simulink model "building_PHPP_v2"  (R2023b)
settings: Solver=ode23s  StartTime=-building.preruntime+8760*3600  StopTime=building.runtime+8760*3600  EnableMultiTasking=on
PreLoadFcn:
  | tic
StartFcn:
  | pre_time = toc
  | assignin('base','pre_time',pre_time)
  | tic
StopFcn:
  | time = toc
  | assignin('base','time',time)
values from neighbouring files (symbols this model uses):
  building = obj    [BUILDING.m]    (also in create_building_automatic.m = building.save(); ini_building_automatic.m = building.add_variant_hvac(building.variant_hvac, hvac); load_building_automatic.m = building.save())
  cp = str2num(value)    [CONSTRUCTION.m]
  p = [timevec_weather weather(:,12)]    [BOUNDARY.m]    (also in WEATHER.m = 0; init_carnotUIBK.m = cell2mat(carnotUIBKpaths(i,2)))
  rho = str2num(value)    [CONSTRUCTION.m]    (also in theta_ground_v1.m = 2000)
undefined symbols (not defined in the file or in its folder): Dreifach, get_building, Qdot_C, Qdot_C_energy, Qdot_H, Qdot_H_energy, Qdot_I_electricity, Qdot_I_electricity_energy, Qdot_I_light, Qdot_I_light_energy, Qdot_I_person, Qdot_I_person_energy, Qdot_S, Qdot_S_energy, Qdot_T_ground, Qdot_T_ground_energy, Qdot_T_neighbour, Qdot_T_neighbour_energy, Qdot_T_opaque, Qdot_T_opaque_energy, Qdot_T_window, Qdot_T_window_energy, Qdot_V_infiltration, Qdot_V_infiltration_energy, Qdot_V_mech, Qdot_V_mech_energy, Qdot_V_window, Qdot_V_window_energy, Tc, Tr, Ts, Wärmeschutzglas, x_CO2, x_H2O, x_VOC
libraries: carnotUIBK x2418, carnot x1
(part 31 of 32)

== system building_PHPP_v2/DATALOGGER/logger_BDB/z1 ==
  BDB : Inport
  Bus Assignment : BusAssignment  AssignedSignals=Qdot_T_opaque_energy,Qdot_T_ground_energy,Qdot_T_neighbour_energy,Qdot_T_window_energy,Qdot_V_mech_energy,Qdot_V_window_energy,Qdot_V_infiltration_energy,Qdot_S_energy,Qdot_I_person_energy,Qdot_I_light_energy,Qdot_I_electricity_energy,Qdot_H_energy,Qdot_C_energy
  Bus Creator1 : BusCreator  Inputs=13
  Bus Selector1 : BusSelector  OutputSignals=z1.Qdot_T_opaque,z1.Qdot_T_ground,z1.Qdot_T_neighbour,z1.Qdot_T_window,z1.Qdot_V_mech,z1.Qdot_V_window,z1.Qdot_V_infiltration,z1.Qdot_S,z1.Qdot_I_person,z1.Qdot_I_light,z1.Qdot_I_electricity,z1.Qdot_H,z1.Qdot_C
  Constant{,1..12} (13 alike) : Constant  Value=0
  Subsystem : Subsystem
  Subsystem1 : Subsystem
  Subsystem10 : Subsystem
  Subsystem11 : Subsystem
  Subsystem12 : Subsystem
  Subsystem2 : Subsystem
  Subsystem3 : Subsystem
  Subsystem4 : Subsystem
  Subsystem5 : Subsystem
  Subsystem6 : Subsystem
  Subsystem7 : Subsystem
  Subsystem8 : Subsystem
  Subsystem9 : Subsystem
  BDBenergy : Outport  VectorParamsAs1DForOutWhenUnconnected=off
  wires:
  Constant12/1 -> Bus Creator1/13  "Qdot_C_energy"
  Constant2/1 -> Bus Creator1/3  "Qdot_T_neighbour_energy"
  Constant4/1 -> Bus Creator1/5  "Qdot_V_mech_energy"
  Constant9/1 -> Bus Creator1/10  "Qdot_I_light_energy"
  Constant1/1 -> Bus Creator1/2  "Qdot_T_ground_energy"
  Constant3/1 -> Bus Creator1/4  "Qdot_T_window_energy"
  Constant11/1 -> Bus Creator1/12  "Qdot_H_energy"
  Constant10/1 -> Bus Creator1/11  "Qdot_I_electricity_energy"
  Constant/1 -> Bus Creator1/1  "Qdot_T_opaque_energy"
  Constant8/1 -> Bus Creator1/8  "Qdot_S_energy"
  Constant7/1 -> Bus Creator1/9  "Qdot_I_person_energy"
  Constant6/1 -> Bus Creator1/7  "Qdot_V_infiltration_energy"
  BDB/1 -> Bus Selector1/1
  Constant5/1 -> Bus Creator1/6  "Qdot_V_window_energy"
  Bus Selector1/1 -> Subsystem/1(In1)  "<Qdot_T_opaque>"
  Bus Selector1/4 -> Subsystem3/1(In1)  "<Qdot_T_window>"
  Bus Selector1/3 -> Subsystem2/1(In1)  "<Qdot_T_neighbour>"
  Bus Selector1/2 -> Subsystem1/1(In1)  "<Qdot_T_ground>"
  Bus Selector1/9 -> Subsystem8/1(In1)  "<Qdot_I_person>"
  Bus Selector1/10 -> Subsystem9/1(In1)  "<Qdot_I_light>"
  Bus Selector1/11 -> Subsystem10/1(In1)  "<Qdot_I_electricity>"
  Bus Selector1/12 -> Subsystem11/1(In1)  "<Qdot_H>"
  Bus Selector1/13 -> Subsystem12/1(In1)  "<Qdot_C>"
  Bus Selector1/8 -> Subsystem7/1(In1)  "<Qdot_S>"
  Bus Selector1/7 -> Subsystem6/1(In1)  "<Qdot_V_infiltration>"
  Bus Selector1/6 -> Subsystem5/1(In1)  "<Qdot_V_window>"
  Bus Selector1/5 -> Subsystem4/1(In1)  "<Qdot_V_mech>"
  Bus Assignment/1 -> BDBenergy/1
  Bus Creator1/1 -> Bus Assignment/1
  Subsystem/1(Out1) -> Bus Assignment/2
  Subsystem12/1(Out1) -> Bus Assignment/14
  Subsystem11/1(Out1) -> Bus Assignment/13
  Subsystem10/1(Out1) -> Bus Assignment/12
  Subsystem9/1(Out1) -> Bus Assignment/11
  Subsystem8/1(Out1) -> Bus Assignment/10
  Subsystem7/1(Out1) -> Bus Assignment/9
  Subsystem6/1(Out1) -> Bus Assignment/8
  Subsystem5/1(Out1) -> Bus Assignment/7
  Subsystem4/1(Out1) -> Bus Assignment/6
  Subsystem3/1(Out1) -> Bus Assignment/5
  Subsystem2/1(Out1) -> Bus Assignment/4
  Subsystem1/1(Out1) -> Bus Assignment/3

== system building_PHPP_v2/DATALOGGER/logger_BDB/z10 ==
  BDB : Inport
  Bus Assignment : BusAssignment  AssignedSignals=Qdot_T_opaque_energy,Qdot_T_ground_energy,Qdot_T_neighbour_energy,Qdot_T_window_energy,Qdot_V_mech_energy,Qdot_V_window_energy,Qdot_V_infiltration_energy,Qdot_S_energy,Qdot_I_person_energy,Qdot_I_light_energy,Qdot_I_electricity_energy,Qdot_H_energy,Qdot_C_energy
  Bus Creator1 : BusCreator  Inputs=13
  Bus Selector1 : BusSelector  OutputSignals=z10.Qdot_T_opaque,z10.Qdot_T_ground,z10.Qdot_T_neighbour,z10.Qdot_T_window,z10.Qdot_V_mech,z10.Qdot_V_window,z10.Qdot_V_infiltration,z10.Qdot_S,z10.Qdot_I_person,z10.Qdot_I_light,z10.Qdot_I_electricity,z10.Qdot_H,z10.Qdot_C
  Constant{,1..12} (13 alike) : Constant  Value=0
  Subsystem : Subsystem
  Subsystem1 : Subsystem
  Subsystem10 : Subsystem
  Subsystem11 : Subsystem
  Subsystem12 : Subsystem
  Subsystem2 : Subsystem
  Subsystem3 : Subsystem
  Subsystem4 : Subsystem
  Subsystem5 : Subsystem
  Subsystem6 : Subsystem
  Subsystem7 : Subsystem
  Subsystem8 : Subsystem
  Subsystem9 : Subsystem
  BDBenergy : Outport  VectorParamsAs1DForOutWhenUnconnected=off
  wires:
  Subsystem1/1(Out1) -> Bus Assignment/3
  Subsystem2/1(Out1) -> Bus Assignment/4
  Subsystem3/1(Out1) -> Bus Assignment/5
  Subsystem4/1(Out1) -> Bus Assignment/6
  Subsystem5/1(Out1) -> Bus Assignment/7
  Subsystem6/1(Out1) -> Bus Assignment/8
  Subsystem7/1(Out1) -> Bus Assignment/9
  Subsystem8/1(Out1) -> Bus Assignment/10
  Subsystem9/1(Out1) -> Bus Assignment/11
  Subsystem10/1(Out1) -> Bus Assignment/12
  Subsystem11/1(Out1) -> Bus Assignment/13
  Subsystem12/1(Out1) -> Bus Assignment/14
  Subsystem/1(Out1) -> Bus Assignment/2
  Bus Creator1/1 -> Bus Assignment/1
  Bus Assignment/1 -> BDBenergy/1
  Bus Selector1/5 -> Subsystem4/1(In1)  "<Qdot_V_mech>"
  Bus Selector1/6 -> Subsystem5/1(In1)  "<Qdot_V_window>"
  Bus Selector1/7 -> Subsystem6/1(In1)  "<Qdot_V_infiltration>"
  Bus Selector1/8 -> Subsystem7/1(In1)  "<Qdot_S>"
  Bus Selector1/13 -> Subsystem12/1(In1)  "<Qdot_C>"
  Bus Selector1/12 -> Subsystem11/1(In1)  "<Qdot_H>"
  Bus Selector1/11 -> Subsystem10/1(In1)  "<Qdot_I_electricity>"
  Bus Selector1/10 -> Subsystem9/1(In1)  "<Qdot_I_light>"
  Bus Selector1/9 -> Subsystem8/1(In1)  "<Qdot_I_person>"
  Bus Selector1/2 -> Subsystem1/1(In1)  "<Qdot_T_ground>"
  Bus Selector1/3 -> Subsystem2/1(In1)  "<Qdot_T_neighbour>"
  Bus Selector1/4 -> Subsystem3/1(In1)  "<Qdot_T_window>"
  Bus Selector1/1 -> Subsystem/1(In1)  "<Qdot_T_opaque>"
  Constant5/1 -> Bus Creator1/6  "Qdot_V_window_energy"
  BDB/1 -> Bus Selector1/1
  Constant6/1 -> Bus Creator1/7  "Qdot_V_infiltration_energy"
  Constant7/1 -> Bus Creator1/9  "Qdot_I_person_energy"
  Constant8/1 -> Bus Creator1/8  "Qdot_S_energy"
  Constant/1 -> Bus Creator1/1  "Qdot_T_opaque_energy"
  Constant10/1 -> Bus Creator1/11  "Qdot_I_electricity_energy"
  Constant11/1 -> Bus Creator1/12  "Qdot_H_energy"
  Constant3/1 -> Bus Creator1/4  "Qdot_T_window_energy"
  Constant1/1 -> Bus Creator1/2  "Qdot_T_ground_energy"
  Constant9/1 -> Bus Creator1/10  "Qdot_I_light_energy"
  Constant4/1 -> Bus Creator1/5  "Qdot_V_mech_energy"
  Constant2/1 -> Bus Creator1/3  "Qdot_T_neighbour_energy"
  Constant12/1 -> Bus Creator1/13  "Qdot_C_energy"

== system building_PHPP_v2/DATALOGGER/logger_BDB/z2 ==
  BDB : Inport
  Bus Assignment : BusAssignment  AssignedSignals=Qdot_T_opaque_energy,Qdot_T_ground_energy,Qdot_T_neighbour_energy,Qdot_T_window_energy,Qdot_V_mech_energy,Qdot_V_window_energy,Qdot_V_infiltration_energy,Qdot_S_energy,Qdot_I_person_energy,Qdot_I_light_energy,Qdot_I_electricity_energy,Qdot_H_energy,Qdot_C_energy
  Bus Creator1 : BusCreator  Inputs=13
  Bus Selector1 : BusSelector  OutputSignals=z2.Qdot_T_opaque,z2.Qdot_T_ground,z2.Qdot_T_neighbour,z2.Qdot_T_window,z2.Qdot_V_mech,z2.Qdot_V_window,z2.Qdot_V_infiltration,z2.Qdot_S,z2.Qdot_I_person,z2.Qdot_I_light,z2.Qdot_I_electricity,z2.Qdot_H,z2.Qdot_C
  Constant{,1..12} (13 alike) : Constant  Value=0
  Subsystem : Subsystem
  Subsystem1 : Subsystem
  Subsystem10 : Subsystem
  Subsystem11 : Subsystem
  Subsystem12 : Subsystem
  Subsystem2 : Subsystem
  Subsystem3 : Subsystem
  Subsystem4 : Subsystem
  Subsystem5 : Subsystem
  Subsystem6 : Subsystem
  Subsystem7 : Subsystem
  Subsystem8 : Subsystem
  Subsystem9 : Subsystem
  BDBenergy : Outport  VectorParamsAs1DForOutWhenUnconnected=off
  wires:
  Subsystem1/1(Out1) -> Bus Assignment/3
  Subsystem2/1(Out1) -> Bus Assignment/4
  Subsystem3/1(Out1) -> Bus Assignment/5
  Subsystem4/1(Out1) -> Bus Assignment/6
  Subsystem5/1(Out1) -> Bus Assignment/7
  Subsystem6/1(Out1) -> Bus Assignment/8
  Subsystem7/1(Out1) -> Bus Assignment/9
  Subsystem8/1(Out1) -> Bus Assignment/10
  Subsystem9/1(Out1) -> Bus Assignment/11
  Subsystem10/1(Out1) -> Bus Assignment/12
  Subsystem11/1(Out1) -> Bus Assignment/13
  Subsystem12/1(Out1) -> Bus Assignment/14
  Subsystem/1(Out1) -> Bus Assignment/2
  Bus Creator1/1 -> Bus Assignment/1
  Bus Assignment/1 -> BDBenergy/1
  Bus Selector1/5 -> Subsystem4/1(In1)  "<Qdot_V_mech>"
  Bus Selector1/6 -> Subsystem5/1(In1)  "<Qdot_V_window>"
  Bus Selector1/7 -> Subsystem6/1(In1)  "<Qdot_V_infiltration>"
  Bus Selector1/8 -> Subsystem7/1(In1)  "<Qdot_S>"
  Bus Selector1/13 -> Subsystem12/1(In1)  "<Qdot_C>"
  Bus Selector1/12 -> Subsystem11/1(In1)  "<Qdot_H>"
  Bus Selector1/11 -> Subsystem10/1(In1)  "<Qdot_I_electricity>"
  Bus Selector1/10 -> Subsystem9/1(In1)  "<Qdot_I_light>"
  Bus Selector1/9 -> Subsystem8/1(In1)  "<Qdot_I_person>"
  Bus Selector1/2 -> Subsystem1/1(In1)  "<Qdot_T_ground>"
  Bus Selector1/3 -> Subsystem2/1(In1)  "<Qdot_T_neighbour>"
  Bus Selector1/4 -> Subsystem3/1(In1)  "<Qdot_T_window>"
  Bus Selector1/1 -> Subsystem/1(In1)  "<Qdot_T_opaque>"
  Constant5/1 -> Bus Creator1/6  "Qdot_V_window_energy"
  BDB/1 -> Bus Selector1/1
  Constant6/1 -> Bus Creator1/7  "Qdot_V_infiltration_energy"
  Constant7/1 -> Bus Creator1/9  "Qdot_I_person_energy"
  Constant8/1 -> Bus Creator1/8  "Qdot_S_energy"
  Constant/1 -> Bus Creator1/1  "Qdot_T_opaque_energy"
  Constant10/1 -> Bus Creator1/11  "Qdot_I_electricity_energy"
  Constant11/1 -> Bus Creator1/12  "Qdot_H_energy"
  Constant3/1 -> Bus Creator1/4  "Qdot_T_window_energy"
  Constant1/1 -> Bus Creator1/2  "Qdot_T_ground_energy"
  Constant9/1 -> Bus Creator1/10  "Qdot_I_light_energy"
  Constant4/1 -> Bus Creator1/5  "Qdot_V_mech_energy"
  Constant2/1 -> Bus Creator1/3  "Qdot_T_neighbour_energy"
  Constant12/1 -> Bus Creator1/13  "Qdot_C_energy"

== system building_PHPP_v2/DATALOGGER/logger_BDB/z3 ==
  BDB : Inport
  Bus Assignment : BusAssignment  AssignedSignals=Qdot_T_opaque_energy,Qdot_T_ground_energy,Qdot_T_neighbour_energy,Qdot_T_window_energy,Qdot_V_mech_energy,Qdot_V_window_energy,Qdot_V_infiltration_energy,Qdot_S_energy,Qdot_I_person_energy,Qdot_I_light_energy,Qdot_I_electricity_energy,Qdot_H_energy,Qdot_C_energy
  Bus Creator1 : BusCreator  Inputs=13
  Bus Selector1 : BusSelector  OutputSignals=z3.Qdot_T_opaque,z3.Qdot_T_ground,z3.Qdot_T_neighbour,z3.Qdot_T_window,z3.Qdot_V_mech,z3.Qdot_V_window,z3.Qdot_V_infiltration,z3.Qdot_S,z3.Qdot_I_person,z3.Qdot_I_light,z3.Qdot_I_electricity,z3.Qdot_H,z3.Qdot_C
  Constant{,1..12} (13 alike) : Constant  Value=0
  Subsystem : Subsystem
  Subsystem1 : Subsystem
  Subsystem10 : Subsystem
  Subsystem11 : Subsystem
  Subsystem12 : Subsystem
  Subsystem2 : Subsystem
  Subsystem3 : Subsystem
  Subsystem4 : Subsystem
  Subsystem5 : Subsystem
  Subsystem6 : Subsystem
  Subsystem7 : Subsystem
  Subsystem8 : Subsystem
  Subsystem9 : Subsystem
  BDBenergy : Outport  VectorParamsAs1DForOutWhenUnconnected=off
  wires:
  Constant12/1 -> Bus Creator1/13  "Qdot_C_energy"
  Constant2/1 -> Bus Creator1/3  "Qdot_T_neighbour_energy"
  Constant4/1 -> Bus Creator1/5  "Qdot_V_mech_energy"
  Constant9/1 -> Bus Creator1/10  "Qdot_I_light_energy"
  Constant1/1 -> Bus Creator1/2  "Qdot_T_ground_energy"
  Constant3/1 -> Bus Creator1/4  "Qdot_T_window_energy"
  Constant11/1 -> Bus Creator1/12  "Qdot_H_energy"
  Constant10/1 -> Bus Creator1/11  "Qdot_I_electricity_energy"
  Constant/1 -> Bus Creator1/1  "Qdot_T_opaque_energy"
  Constant8/1 -> Bus Creator1/8  "Qdot_S_energy"
  Constant7/1 -> Bus Creator1/9  "Qdot_I_person_energy"
  Constant6/1 -> Bus Creator1/7  "Qdot_V_infiltration_energy"
  BDB/1 -> Bus Selector1/1
  Constant5/1 -> Bus Creator1/6  "Qdot_V_window_energy"
  Bus Selector1/1 -> Subsystem/1(In1)  "<Qdot_T_opaque>"
  Bus Selector1/4 -> Subsystem3/1(In1)  "<Qdot_T_window>"
  Bus Selector1/3 -> Subsystem2/1(In1)  "<Qdot_T_neighbour>"
  Bus Selector1/2 -> Subsystem1/1(In1)  "<Qdot_T_ground>"
  Bus Selector1/9 -> Subsystem8/1(In1)  "<Qdot_I_person>"
  Bus Selector1/10 -> Subsystem9/1(In1)  "<Qdot_I_light>"
  Bus Selector1/11 -> Subsystem10/1(In1)  "<Qdot_I_electricity>"
  Bus Selector1/12 -> Subsystem11/1(In1)  "<Qdot_H>"
  Bus Selector1/13 -> Subsystem12/1(In1)  "<Qdot_C>"
  Bus Selector1/8 -> Subsystem7/1(In1)  "<Qdot_S>"
  Bus Selector1/7 -> Subsystem6/1(In1)  "<Qdot_V_infiltration>"
  Bus Selector1/6 -> Subsystem5/1(In1)  "<Qdot_V_window>"
  Bus Selector1/5 -> Subsystem4/1(In1)  "<Qdot_V_mech>"
  Bus Assignment/1 -> BDBenergy/1
  Bus Creator1/1 -> Bus Assignment/1
  Subsystem/1(Out1) -> Bus Assignment/2
  Subsystem12/1(Out1) -> Bus Assignment/14
  Subsystem11/1(Out1) -> Bus Assignment/13
  Subsystem10/1(Out1) -> Bus Assignment/12
  Subsystem9/1(Out1) -> Bus Assignment/11
  Subsystem8/1(Out1) -> Bus Assignment/10
  Subsystem7/1(Out1) -> Bus Assignment/9
  Subsystem6/1(Out1) -> Bus Assignment/8
  Subsystem5/1(Out1) -> Bus Assignment/7
  Subsystem4/1(Out1) -> Bus Assignment/6
  Subsystem3/1(Out1) -> Bus Assignment/5
  Subsystem2/1(Out1) -> Bus Assignment/4
  Subsystem1/1(Out1) -> Bus Assignment/3

== system building_PHPP_v2/DATALOGGER/logger_BDB/z4 ==
  BDB : Inport
  Bus Assignment : BusAssignment  AssignedSignals=Qdot_T_opaque_energy,Qdot_T_ground_energy,Qdot_T_neighbour_energy,Qdot_T_window_energy,Qdot_V_mech_energy,Qdot_V_window_energy,Qdot_V_infiltration_energy,Qdot_S_energy,Qdot_I_person_energy,Qdot_I_light_energy,Qdot_I_electricity_energy,Qdot_H_energy,Qdot_C_energy
  Bus Creator1 : BusCreator  Inputs=13
  Bus Selector1 : BusSelector  OutputSignals=z4.Qdot_T_opaque,z4.Qdot_T_ground,z4.Qdot_T_neighbour,z4.Qdot_T_window,z4.Qdot_V_mech,z4.Qdot_V_window,z4.Qdot_V_infiltration,z4.Qdot_S,z4.Qdot_I_person,z4.Qdot_I_light,z4.Qdot_I_electricity,z4.Qdot_H,z4.Qdot_C
  Constant{,1..12} (13 alike) : Constant  Value=0
  Subsystem : Subsystem
  Subsystem1 : Subsystem
  Subsystem10 : Subsystem
  Subsystem11 : Subsystem
  Subsystem12 : Subsystem
  Subsystem2 : Subsystem
  Subsystem3 : Subsystem
  Subsystem4 : Subsystem
  Subsystem5 : Subsystem
  Subsystem6 : Subsystem
  Subsystem7 : Subsystem
  Subsystem8 : Subsystem
  Subsystem9 : Subsystem
  BDBenergy : Outport  VectorParamsAs1DForOutWhenUnconnected=off
  wires:
  Subsystem1/1(Out1) -> Bus Assignment/3
  Subsystem2/1(Out1) -> Bus Assignment/4
  Subsystem3/1(Out1) -> Bus Assignment/5
  Subsystem4/1(Out1) -> Bus Assignment/6
  Subsystem5/1(Out1) -> Bus Assignment/7
  Subsystem6/1(Out1) -> Bus Assignment/8
  Subsystem7/1(Out1) -> Bus Assignment/9
  Subsystem8/1(Out1) -> Bus Assignment/10
  Subsystem9/1(Out1) -> Bus Assignment/11
  Subsystem10/1(Out1) -> Bus Assignment/12
  Subsystem11/1(Out1) -> Bus Assignment/13
  Subsystem12/1(Out1) -> Bus Assignment/14
  Subsystem/1(Out1) -> Bus Assignment/2
  Bus Creator1/1 -> Bus Assignment/1
  Bus Assignment/1 -> BDBenergy/1
  Bus Selector1/5 -> Subsystem4/1(In1)  "<Qdot_V_mech>"
  Bus Selector1/6 -> Subsystem5/1(In1)  "<Qdot_V_window>"
  Bus Selector1/7 -> Subsystem6/1(In1)  "<Qdot_V_infiltration>"
  Bus Selector1/8 -> Subsystem7/1(In1)  "<Qdot_S>"
  Bus Selector1/13 -> Subsystem12/1(In1)  "<Qdot_C>"
  Bus Selector1/12 -> Subsystem11/1(In1)  "<Qdot_H>"
  Bus Selector1/11 -> Subsystem10/1(In1)  "<Qdot_I_electricity>"
  Bus Selector1/10 -> Subsystem9/1(In1)  "<Qdot_I_light>"
  Bus Selector1/9 -> Subsystem8/1(In1)  "<Qdot_I_person>"
  Bus Selector1/2 -> Subsystem1/1(In1)  "<Qdot_T_ground>"
  Bus Selector1/3 -> Subsystem2/1(In1)  "<Qdot_T_neighbour>"
  Bus Selector1/4 -> Subsystem3/1(In1)  "<Qdot_T_window>"
  Bus Selector1/1 -> Subsystem/1(In1)  "<Qdot_T_opaque>"
  Constant5/1 -> Bus Creator1/6  "Qdot_V_window_energy"
  BDB/1 -> Bus Selector1/1
  Constant6/1 -> Bus Creator1/7  "Qdot_V_infiltration_energy"
  Constant7/1 -> Bus Creator1/9  "Qdot_I_person_energy"
  Constant8/1 -> Bus Creator1/8  "Qdot_S_energy"
  Constant/1 -> Bus Creator1/1  "Qdot_T_opaque_energy"
  Constant10/1 -> Bus Creator1/11  "Qdot_I_electricity_energy"
  Constant11/1 -> Bus Creator1/12  "Qdot_H_energy"
  Constant3/1 -> Bus Creator1/4  "Qdot_T_window_energy"
  Constant1/1 -> Bus Creator1/2  "Qdot_T_ground_energy"
  Constant9/1 -> Bus Creator1/10  "Qdot_I_light_energy"
  Constant4/1 -> Bus Creator1/5  "Qdot_V_mech_energy"
  Constant2/1 -> Bus Creator1/3  "Qdot_T_neighbour_energy"
  Constant12/1 -> Bus Creator1/13  "Qdot_C_energy"

== system building_PHPP_v2/DATALOGGER/logger_BDB/z5 ==
  BDB : Inport
  Bus Assignment : BusAssignment  AssignedSignals=Qdot_T_opaque_energy,Qdot_T_ground_energy,Qdot_T_neighbour_energy,Qdot_T_window_energy,Qdot_V_mech_energy,Qdot_V_window_energy,Qdot_V_infiltration_energy,Qdot_S_energy,Qdot_I_person_energy,Qdot_I_light_energy,Qdot_I_electricity_energy,Qdot_H_energy,Qdot_C_energy
  Bus Creator1 : BusCreator  Inputs=13
  Bus Selector1 : BusSelector  OutputSignals=z5.Qdot_T_opaque,z5.Qdot_T_ground,z5.Qdot_T_neighbour,z5.Qdot_T_window,z5.Qdot_V_mech,z5.Qdot_V_window,z5.Qdot_V_infiltration,z5.Qdot_S,z5.Qdot_I_person,z5.Qdot_I_light,z5.Qdot_I_electricity,z5.Qdot_H,z5.Qdot_C
  Constant{,1..12} (13 alike) : Constant  Value=0
  Subsystem : Subsystem
  Subsystem1 : Subsystem
  Subsystem10 : Subsystem
  Subsystem11 : Subsystem
  Subsystem12 : Subsystem
  Subsystem2 : Subsystem
  Subsystem3 : Subsystem
  Subsystem4 : Subsystem
  Subsystem5 : Subsystem
  Subsystem6 : Subsystem
  Subsystem7 : Subsystem
  Subsystem8 : Subsystem
  Subsystem9 : Subsystem
  BDBenergy : Outport  VectorParamsAs1DForOutWhenUnconnected=off
  wires:
  Constant12/1 -> Bus Creator1/13  "Qdot_C_energy"
  Constant2/1 -> Bus Creator1/3  "Qdot_T_neighbour_energy"
  Constant4/1 -> Bus Creator1/5  "Qdot_V_mech_energy"
  Constant9/1 -> Bus Creator1/10  "Qdot_I_light_energy"
  Constant1/1 -> Bus Creator1/2  "Qdot_T_ground_energy"
  Constant3/1 -> Bus Creator1/4  "Qdot_T_window_energy"
  Constant11/1 -> Bus Creator1/12  "Qdot_H_energy"
  Constant10/1 -> Bus Creator1/11  "Qdot_I_electricity_energy"
  Constant/1 -> Bus Creator1/1  "Qdot_T_opaque_energy"
  Constant8/1 -> Bus Creator1/8  "Qdot_S_energy"
  Constant7/1 -> Bus Creator1/9  "Qdot_I_person_energy"
  Constant6/1 -> Bus Creator1/7  "Qdot_V_infiltration_energy"
  BDB/1 -> Bus Selector1/1
  Constant5/1 -> Bus Creator1/6  "Qdot_V_window_energy"
  Bus Selector1/1 -> Subsystem/1(In1)  "<Qdot_T_opaque>"
  Bus Selector1/4 -> Subsystem3/1(In1)  "<Qdot_T_window>"
  Bus Selector1/3 -> Subsystem2/1(In1)  "<Qdot_T_neighbour>"
  Bus Selector1/2 -> Subsystem1/1(In1)  "<Qdot_T_ground>"
  Bus Selector1/9 -> Subsystem8/1(In1)  "<Qdot_I_person>"
  Bus Selector1/10 -> Subsystem9/1(In1)  "<Qdot_I_light>"
  Bus Selector1/11 -> Subsystem10/1(In1)  "<Qdot_I_electricity>"
  Bus Selector1/12 -> Subsystem11/1(In1)  "<Qdot_H>"
  Bus Selector1/13 -> Subsystem12/1(In1)  "<Qdot_C>"
  Bus Selector1/8 -> Subsystem7/1(In1)  "<Qdot_S>"
  Bus Selector1/7 -> Subsystem6/1(In1)  "<Qdot_V_infiltration>"
  Bus Selector1/6 -> Subsystem5/1(In1)  "<Qdot_V_window>"
  Bus Selector1/5 -> Subsystem4/1(In1)  "<Qdot_V_mech>"
  Bus Assignment/1 -> BDBenergy/1
  Bus Creator1/1 -> Bus Assignment/1
  Subsystem/1(Out1) -> Bus Assignment/2
  Subsystem12/1(Out1) -> Bus Assignment/14
  Subsystem11/1(Out1) -> Bus Assignment/13
  Subsystem10/1(Out1) -> Bus Assignment/12
  Subsystem9/1(Out1) -> Bus Assignment/11
  Subsystem8/1(Out1) -> Bus Assignment/10
  Subsystem7/1(Out1) -> Bus Assignment/9
  Subsystem6/1(Out1) -> Bus Assignment/8
  Subsystem5/1(Out1) -> Bus Assignment/7
  Subsystem4/1(Out1) -> Bus Assignment/6
  Subsystem3/1(Out1) -> Bus Assignment/5
  Subsystem2/1(Out1) -> Bus Assignment/4
  Subsystem1/1(Out1) -> Bus Assignment/3

== system building_PHPP_v2/DATALOGGER/logger_BDB/z6 ==
  BDB : Inport
  Bus Assignment : BusAssignment  AssignedSignals=Qdot_T_opaque_energy,Qdot_T_ground_energy,Qdot_T_neighbour_energy,Qdot_T_window_energy,Qdot_V_mech_energy,Qdot_V_window_energy,Qdot_V_infiltration_energy,Qdot_S_energy,Qdot_I_person_energy,Qdot_I_light_energy,Qdot_I_electricity_energy,Qdot_H_energy,Qdot_C_energy
  Bus Creator1 : BusCreator  Inputs=13
  Bus Selector1 : BusSelector  OutputSignals=z6.Qdot_T_opaque,z6.Qdot_T_ground,z6.Qdot_T_neighbour,z6.Qdot_T_window,z6.Qdot_V_mech,z6.Qdot_V_window,z6.Qdot_V_infiltration,z6.Qdot_S,z6.Qdot_I_person,z6.Qdot_I_light,z6.Qdot_I_electricity,z6.Qdot_H,z6.Qdot_C
  Constant{,1..12} (13 alike) : Constant  Value=0
  Subsystem : Subsystem
  Subsystem1 : Subsystem
  Subsystem10 : Subsystem
  Subsystem11 : Subsystem
  Subsystem12 : Subsystem
  Subsystem2 : Subsystem
  Subsystem3 : Subsystem
  Subsystem4 : Subsystem
  Subsystem5 : Subsystem
  Subsystem6 : Subsystem
  Subsystem7 : Subsystem
  Subsystem8 : Subsystem
  Subsystem9 : Subsystem
  BDBenergy : Outport  VectorParamsAs1DForOutWhenUnconnected=off
  wires:
  Subsystem1/1(Out1) -> Bus Assignment/3
  Subsystem2/1(Out1) -> Bus Assignment/4
  Subsystem3/1(Out1) -> Bus Assignment/5
  Subsystem4/1(Out1) -> Bus Assignment/6
  Subsystem5/1(Out1) -> Bus Assignment/7
  Subsystem6/1(Out1) -> Bus Assignment/8
  Subsystem7/1(Out1) -> Bus Assignment/9
  Subsystem8/1(Out1) -> Bus Assignment/10
  Subsystem9/1(Out1) -> Bus Assignment/11
  Subsystem10/1(Out1) -> Bus Assignment/12
  Subsystem11/1(Out1) -> Bus Assignment/13
  Subsystem12/1(Out1) -> Bus Assignment/14
  Subsystem/1(Out1) -> Bus Assignment/2
  Bus Creator1/1 -> Bus Assignment/1
  Bus Assignment/1 -> BDBenergy/1
  Bus Selector1/5 -> Subsystem4/1(In1)  "<Qdot_V_mech>"
  Bus Selector1/6 -> Subsystem5/1(In1)  "<Qdot_V_window>"
  Bus Selector1/7 -> Subsystem6/1(In1)  "<Qdot_V_infiltration>"
  Bus Selector1/8 -> Subsystem7/1(In1)  "<Qdot_S>"
  Bus Selector1/13 -> Subsystem12/1(In1)  "<Qdot_C>"
  Bus Selector1/12 -> Subsystem11/1(In1)  "<Qdot_H>"
  Bus Selector1/11 -> Subsystem10/1(In1)  "<Qdot_I_electricity>"
  Bus Selector1/10 -> Subsystem9/1(In1)  "<Qdot_I_light>"
  Bus Selector1/9 -> Subsystem8/1(In1)  "<Qdot_I_person>"
  Bus Selector1/2 -> Subsystem1/1(In1)  "<Qdot_T_ground>"
  Bus Selector1/3 -> Subsystem2/1(In1)  "<Qdot_T_neighbour>"
  Bus Selector1/4 -> Subsystem3/1(In1)  "<Qdot_T_window>"
  Bus Selector1/1 -> Subsystem/1(In1)  "<Qdot_T_opaque>"
  Constant5/1 -> Bus Creator1/6  "Qdot_V_window_energy"
  BDB/1 -> Bus Selector1/1
  Constant6/1 -> Bus Creator1/7  "Qdot_V_infiltration_energy"
  Constant7/1 -> Bus Creator1/9  "Qdot_I_person_energy"
  Constant8/1 -> Bus Creator1/8  "Qdot_S_energy"
  Constant/1 -> Bus Creator1/1  "Qdot_T_opaque_energy"
  Constant10/1 -> Bus Creator1/11  "Qdot_I_electricity_energy"
  Constant11/1 -> Bus Creator1/12  "Qdot_H_energy"
  Constant3/1 -> Bus Creator1/4  "Qdot_T_window_energy"
  Constant1/1 -> Bus Creator1/2  "Qdot_T_ground_energy"
  Constant9/1 -> Bus Creator1/10  "Qdot_I_light_energy"
  Constant4/1 -> Bus Creator1/5  "Qdot_V_mech_energy"
  Constant2/1 -> Bus Creator1/3  "Qdot_T_neighbour_energy"
  Constant12/1 -> Bus Creator1/13  "Qdot_C_energy"

== system building_PHPP_v2/DATALOGGER/logger_BDB/z7 ==
  BDB : Inport
  Bus Assignment : BusAssignment  AssignedSignals=Qdot_T_opaque_energy,Qdot_T_ground_energy,Qdot_T_neighbour_energy,Qdot_T_window_energy,Qdot_V_mech_energy,Qdot_V_window_energy,Qdot_V_infiltration_energy,Qdot_S_energy,Qdot_I_person_energy,Qdot_I_light_energy,Qdot_I_electricity_energy,Qdot_H_energy,Qdot_C_energy
  Bus Creator1 : BusCreator  Inputs=13
  Bus Selector1 : BusSelector  OutputSignals=z7.Qdot_T_opaque,z7.Qdot_T_ground,z7.Qdot_T_neighbour,z7.Qdot_T_window,z7.Qdot_V_mech,z7.Qdot_V_window,z7.Qdot_V_infiltration,z7.Qdot_S,z7.Qdot_I_person,z7.Qdot_I_light,z7.Qdot_I_electricity,z7.Qdot_H,z7.Qdot_C
  Constant{,1..12} (13 alike) : Constant  Value=0
  Subsystem : Subsystem
  Subsystem1 : Subsystem
  Subsystem10 : Subsystem
  Subsystem11 : Subsystem
  Subsystem12 : Subsystem
  Subsystem2 : Subsystem
  Subsystem3 : Subsystem
  Subsystem4 : Subsystem
  Subsystem5 : Subsystem
  Subsystem6 : Subsystem
  Subsystem7 : Subsystem
  Subsystem8 : Subsystem
  Subsystem9 : Subsystem
  BDBenergy : Outport  VectorParamsAs1DForOutWhenUnconnected=off
  wires:
  Constant12/1 -> Bus Creator1/13  "Qdot_C_energy"
  Constant2/1 -> Bus Creator1/3  "Qdot_T_neighbour_energy"
  Constant4/1 -> Bus Creator1/5  "Qdot_V_mech_energy"
  Constant9/1 -> Bus Creator1/10  "Qdot_I_light_energy"
  Constant1/1 -> Bus Creator1/2  "Qdot_T_ground_energy"
  Constant3/1 -> Bus Creator1/4  "Qdot_T_window_energy"
  Constant11/1 -> Bus Creator1/12  "Qdot_H_energy"
  Constant10/1 -> Bus Creator1/11  "Qdot_I_electricity_energy"
  Constant/1 -> Bus Creator1/1  "Qdot_T_opaque_energy"
  Constant8/1 -> Bus Creator1/8  "Qdot_S_energy"
  Constant7/1 -> Bus Creator1/9  "Qdot_I_person_energy"
  Constant6/1 -> Bus Creator1/7  "Qdot_V_infiltration_energy"
  BDB/1 -> Bus Selector1/1
  Constant5/1 -> Bus Creator1/6  "Qdot_V_window_energy"
  Bus Selector1/1 -> Subsystem/1(In1)  "<Qdot_T_opaque>"
  Bus Selector1/4 -> Subsystem3/1(In1)  "<Qdot_T_window>"
  Bus Selector1/3 -> Subsystem2/1(In1)  "<Qdot_T_neighbour>"
  Bus Selector1/2 -> Subsystem1/1(In1)  "<Qdot_T_ground>"
  Bus Selector1/9 -> Subsystem8/1(In1)  "<Qdot_I_person>"
  Bus Selector1/10 -> Subsystem9/1(In1)  "<Qdot_I_light>"
  Bus Selector1/11 -> Subsystem10/1(In1)  "<Qdot_I_electricity>"
  Bus Selector1/12 -> Subsystem11/1(In1)  "<Qdot_H>"
  Bus Selector1/13 -> Subsystem12/1(In1)  "<Qdot_C>"
  Bus Selector1/8 -> Subsystem7/1(In1)  "<Qdot_S>"
  Bus Selector1/7 -> Subsystem6/1(In1)  "<Qdot_V_infiltration>"
  Bus Selector1/6 -> Subsystem5/1(In1)  "<Qdot_V_window>"
  Bus Selector1/5 -> Subsystem4/1(In1)  "<Qdot_V_mech>"
  Bus Assignment/1 -> BDBenergy/1
  Bus Creator1/1 -> Bus Assignment/1
  Subsystem/1(Out1) -> Bus Assignment/2
  Subsystem12/1(Out1) -> Bus Assignment/14
  Subsystem11/1(Out1) -> Bus Assignment/13
  Subsystem10/1(Out1) -> Bus Assignment/12
  Subsystem9/1(Out1) -> Bus Assignment/11
  Subsystem8/1(Out1) -> Bus Assignment/10
  Subsystem7/1(Out1) -> Bus Assignment/9
  Subsystem6/1(Out1) -> Bus Assignment/8
  Subsystem5/1(Out1) -> Bus Assignment/7
  Subsystem4/1(Out1) -> Bus Assignment/6
  Subsystem3/1(Out1) -> Bus Assignment/5
  Subsystem2/1(Out1) -> Bus Assignment/4
  Subsystem1/1(Out1) -> Bus Assignment/3

== system building_PHPP_v2/DATALOGGER/logger_BDB/z8 ==
  BDB : Inport
  Bus Assignment : BusAssignment  AssignedSignals=Qdot_T_opaque_energy,Qdot_T_ground_energy,Qdot_T_neighbour_energy,Qdot_T_window_energy,Qdot_V_mech_energy,Qdot_V_window_energy,Qdot_V_infiltration_energy,Qdot_S_energy,Qdot_I_person_energy,Qdot_I_light_energy,Qdot_I_electricity_energy,Qdot_H_energy,Qdot_C_energy
  Bus Creator1 : BusCreator  Inputs=13
  Bus Selector1 : BusSelector  OutputSignals=z8.Qdot_T_opaque,z8.Qdot_T_ground,z8.Qdot_T_neighbour,z8.Qdot_T_window,z8.Qdot_V_mech,z8.Qdot_V_window,z8.Qdot_V_infiltration,z8.Qdot_S,z8.Qdot_I_person,z8.Qdot_I_light,z8.Qdot_I_electricity,z8.Qdot_H,z8.Qdot_C
  Constant{,1..12} (13 alike) : Constant  Value=0
  Subsystem : Subsystem
  Subsystem1 : Subsystem
  Subsystem10 : Subsystem
  Subsystem11 : Subsystem
  Subsystem12 : Subsystem
  Subsystem2 : Subsystem
  Subsystem3 : Subsystem
  Subsystem4 : Subsystem
  Subsystem5 : Subsystem
  Subsystem6 : Subsystem
  Subsystem7 : Subsystem
  Subsystem8 : Subsystem
  Subsystem9 : Subsystem
  BDBenergy : Outport  VectorParamsAs1DForOutWhenUnconnected=off
  wires:
  Subsystem1/1(Out1) -> Bus Assignment/3
  Subsystem2/1(Out1) -> Bus Assignment/4
  Subsystem3/1(Out1) -> Bus Assignment/5
  Subsystem4/1(Out1) -> Bus Assignment/6
  Subsystem5/1(Out1) -> Bus Assignment/7
  Subsystem6/1(Out1) -> Bus Assignment/8
  Subsystem7/1(Out1) -> Bus Assignment/9
  Subsystem8/1(Out1) -> Bus Assignment/10
  Subsystem9/1(Out1) -> Bus Assignment/11
  Subsystem10/1(Out1) -> Bus Assignment/12
  Subsystem11/1(Out1) -> Bus Assignment/13
  Subsystem12/1(Out1) -> Bus Assignment/14
  Subsystem/1(Out1) -> Bus Assignment/2
  Bus Creator1/1 -> Bus Assignment/1
  Bus Assignment/1 -> BDBenergy/1
  Bus Selector1/5 -> Subsystem4/1(In1)  "<Qdot_V_mech>"
  Bus Selector1/6 -> Subsystem5/1(In1)  "<Qdot_V_window>"
  Bus Selector1/7 -> Subsystem6/1(In1)  "<Qdot_V_infiltration>"
  Bus Selector1/8 -> Subsystem7/1(In1)  "<Qdot_S>"
  Bus Selector1/13 -> Subsystem12/1(In1)  "<Qdot_C>"
  Bus Selector1/12 -> Subsystem11/1(In1)  "<Qdot_H>"
  Bus Selector1/11 -> Subsystem10/1(In1)  "<Qdot_I_electricity>"
  Bus Selector1/10 -> Subsystem9/1(In1)  "<Qdot_I_light>"
  Bus Selector1/9 -> Subsystem8/1(In1)  "<Qdot_I_person>"
  Bus Selector1/2 -> Subsystem1/1(In1)  "<Qdot_T_ground>"
  Bus Selector1/3 -> Subsystem2/1(In1)  "<Qdot_T_neighbour>"
  Bus Selector1/4 -> Subsystem3/1(In1)  "<Qdot_T_window>"
  Bus Selector1/1 -> Subsystem/1(In1)  "<Qdot_T_opaque>"
  Constant5/1 -> Bus Creator1/6  "Qdot_V_window_energy"
  BDB/1 -> Bus Selector1/1
  Constant6/1 -> Bus Creator1/7  "Qdot_V_infiltration_energy"
  Constant7/1 -> Bus Creator1/9  "Qdot_I_person_energy"
  Constant8/1 -> Bus Creator1/8  "Qdot_S_energy"
  Constant/1 -> Bus Creator1/1  "Qdot_T_opaque_energy"
  Constant10/1 -> Bus Creator1/11  "Qdot_I_electricity_energy"
  Constant11/1 -> Bus Creator1/12  "Qdot_H_energy"
  Constant3/1 -> Bus Creator1/4  "Qdot_T_window_energy"
  Constant1/1 -> Bus Creator1/2  "Qdot_T_ground_energy"
  Constant9/1 -> Bus Creator1/10  "Qdot_I_light_energy"
  Constant4/1 -> Bus Creator1/5  "Qdot_V_mech_energy"
  Constant2/1 -> Bus Creator1/3  "Qdot_T_neighbour_energy"
  Constant12/1 -> Bus Creator1/13  "Qdot_C_energy"

== system building_PHPP_v2/DATALOGGER/logger_BDB/z9 ==
  BDB : Inport
  Bus Assignment : BusAssignment  AssignedSignals=Qdot_T_opaque_energy,Qdot_T_ground_energy,Qdot_T_neighbour_energy,Qdot_T_window_energy,Qdot_V_mech_energy,Qdot_V_window_energy,Qdot_V_infiltration_energy,Qdot_S_energy,Qdot_I_person_energy,Qdot_I_light_energy,Qdot_I_electricity_energy,Qdot_H_energy,Qdot_C_energy
  Bus Creator1 : BusCreator  Inputs=13
  Bus Selector1 : BusSelector  OutputSignals=z9.Qdot_T_opaque,z9.Qdot_T_ground,z9.Qdot_T_neighbour,z9.Qdot_T_window,z9.Qdot_V_mech,z9.Qdot_V_window,z9.Qdot_V_infiltration,z9.Qdot_S,z9.Qdot_I_person,z9.Qdot_I_light,z9.Qdot_I_electricity,z9.Qdot_H,z9.Qdot_C
  Constant{,1..12} (13 alike) : Constant  Value=0
  Subsystem : Subsystem
  Subsystem1 : Subsystem
  Subsystem10 : Subsystem
  Subsystem11 : Subsystem
  Subsystem12 : Subsystem
  Subsystem2 : Subsystem
  Subsystem3 : Subsystem
  Subsystem4 : Subsystem
  Subsystem5 : Subsystem
  Subsystem6 : Subsystem
  Subsystem7 : Subsystem
  Subsystem8 : Subsystem
  Subsystem9 : Subsystem
  BDBenergy : Outport  VectorParamsAs1DForOutWhenUnconnected=off
  wires:
  Constant12/1 -> Bus Creator1/13  "Qdot_C_energy"
  Constant2/1 -> Bus Creator1/3  "Qdot_T_neighbour_energy"
  Constant4/1 -> Bus Creator1/5  "Qdot_V_mech_energy"
  Constant9/1 -> Bus Creator1/10  "Qdot_I_light_energy"
  Constant1/1 -> Bus Creator1/2  "Qdot_T_ground_energy"
  Constant3/1 -> Bus Creator1/4  "Qdot_T_window_energy"
  Constant11/1 -> Bus Creator1/12  "Qdot_H_energy"
  Constant10/1 -> Bus Creator1/11  "Qdot_I_electricity_energy"
  Constant/1 -> Bus Creator1/1  "Qdot_T_opaque_energy"
  Constant8/1 -> Bus Creator1/8  "Qdot_S_energy"
  Constant7/1 -> Bus Creator1/9  "Qdot_I_person_energy"
  Constant6/1 -> Bus Creator1/7  "Qdot_V_infiltration_energy"
  BDB/1 -> Bus Selector1/1
  Constant5/1 -> Bus Creator1/6  "Qdot_V_window_energy"
  Bus Selector1/1 -> Subsystem/1(In1)  "<Qdot_T_opaque>"
  Bus Selector1/4 -> Subsystem3/1(In1)  "<Qdot_T_window>"
  Bus Selector1/3 -> Subsystem2/1(In1)  "<Qdot_T_neighbour>"
  Bus Selector1/2 -> Subsystem1/1(In1)  "<Qdot_T_ground>"
  Bus Selector1/9 -> Subsystem8/1(In1)  "<Qdot_I_person>"
  Bus Selector1/10 -> Subsystem9/1(In1)  "<Qdot_I_light>"
  Bus Selector1/11 -> Subsystem10/1(In1)  "<Qdot_I_electricity>"
  Bus Selector1/12 -> Subsystem11/1(In1)  "<Qdot_H>"
  Bus Selector1/13 -> Subsystem12/1(In1)  "<Qdot_C>"
  Bus Selector1/8 -> Subsystem7/1(In1)  "<Qdot_S>"
  Bus Selector1/7 -> Subsystem6/1(In1)  "<Qdot_V_infiltration>"
  Bus Selector1/6 -> Subsystem5/1(In1)  "<Qdot_V_window>"
  Bus Selector1/5 -> Subsystem4/1(In1)  "<Qdot_V_mech>"
  Bus Assignment/1 -> BDBenergy/1
  Bus Creator1/1 -> Bus Assignment/1
  Subsystem/1(Out1) -> Bus Assignment/2
  Subsystem12/1(Out1) -> Bus Assignment/14
  Subsystem11/1(Out1) -> Bus Assignment/13
  Subsystem10/1(Out1) -> Bus Assignment/12
  Subsystem9/1(Out1) -> Bus Assignment/11
  Subsystem8/1(Out1) -> Bus Assignment/10
  Subsystem7/1(Out1) -> Bus Assignment/9
  Subsystem6/1(Out1) -> Bus Assignment/8
  Subsystem5/1(Out1) -> Bus Assignment/7
  Subsystem4/1(Out1) -> Bus Assignment/6
  Subsystem3/1(Out1) -> Bus Assignment/5
  Subsystem2/1(Out1) -> Bus Assignment/4
  Subsystem1/1(Out1) -> Bus Assignment/3

== system building_PHPP_v2/DATALOGGER/logger_BDB/z1/Subsystem ==
  In1 : Inport
  Integrator1 : Integrator
  Ws->kWh : Gain  Gain=1/3600/1000
  Out1 : Outport  VectorParamsAs1DForOutWhenUnconnected=off
  wires:
  Ws->kWh/1 -> Out1/1
  Integrator1/1 -> Ws->kWh/1
  In1/1 -> Integrator1/1

== system building_PHPP_v2/DATALOGGER/logger_BDB/z1/Subsystem1 ==
  In1 : Inport
  Integrator1 : Integrator
  Ws->kWh : Gain  Gain=1/3600/1000
  Out1 : Outport  VectorParamsAs1DForOutWhenUnconnected=off
  wires:
  In1/1 -> Integrator1/1
  Integrator1/1 -> Ws->kWh/1
  Ws->kWh/1 -> Out1/1

== system building_PHPP_v2/DATALOGGER/logger_BDB/z1/Subsystem10 ==
  In1 : Inport
  Integrator1 : Integrator
  Ws->kWh : Gain  Gain=1/3600/1000
  Out1 : Outport  VectorParamsAs1DForOutWhenUnconnected=off
  wires:
  Ws->kWh/1 -> Out1/1
  Integrator1/1 -> Ws->kWh/1
  In1/1 -> Integrator1/1

== system building_PHPP_v2/DATALOGGER/logger_BDB/z1/Subsystem11 ==
  In1 : Inport
  Integrator1 : Integrator
  Ws->kWh : Gain  Gain=1/3600/1000
  Out1 : Outport  VectorParamsAs1DForOutWhenUnconnected=off
  wires:
  In1/1 -> Integrator1/1
  Integrator1/1 -> Ws->kWh/1
  Ws->kWh/1 -> Out1/1

== system building_PHPP_v2/DATALOGGER/logger_BDB/z1/Subsystem12 ==
  In1 : Inport
  Integrator1 : Integrator
  Ws->kWh : Gain  Gain=1/3600/1000
  Out1 : Outport  VectorParamsAs1DForOutWhenUnconnected=off
  wires:
  Ws->kWh/1 -> Out1/1
  Integrator1/1 -> Ws->kWh/1
  In1/1 -> Integrator1/1

== system building_PHPP_v2/DATALOGGER/logger_BDB/z1/Subsystem2 ==
  In1 : Inport
  Integrator1 : Integrator
  Ws->kWh : Gain  Gain=1/3600/1000
  Out1 : Outport  VectorParamsAs1DForOutWhenUnconnected=off
  wires:
  Ws->kWh/1 -> Out1/1
  Integrator1/1 -> Ws->kWh/1
  In1/1 -> Integrator1/1

== system building_PHPP_v2/DATALOGGER/logger_BDB/z1/Subsystem3 ==
  In1 : Inport
  Integrator1 : Integrator
  Ws->kWh : Gain  Gain=1/3600/1000
  Out1 : Outport  VectorParamsAs1DForOutWhenUnconnected=off
  wires:
  In1/1 -> Integrator1/1
  Integrator1/1 -> Ws->kWh/1
  Ws->kWh/1 -> Out1/1

== system building_PHPP_v2/DATALOGGER/logger_BDB/z1/Subsystem4 ==
  In1 : Inport
  Integrator1 : Integrator
  Ws->kWh : Gain  Gain=1/3600/1000
  Out1 : Outport  VectorParamsAs1DForOutWhenUnconnected=off
  wires:
  Ws->kWh/1 -> Out1/1
  Integrator1/1 -> Ws->kWh/1
  In1/1 -> Integrator1/1

== system building_PHPP_v2/DATALOGGER/logger_BDB/z1/Subsystem5 ==
  In1 : Inport
  Integrator1 : Integrator
  Ws->kWh : Gain  Gain=1/3600/1000
  Out1 : Outport  VectorParamsAs1DForOutWhenUnconnected=off
  wires:
  In1/1 -> Integrator1/1
  Integrator1/1 -> Ws->kWh/1
  Ws->kWh/1 -> Out1/1

== system building_PHPP_v2/DATALOGGER/logger_BDB/z1/Subsystem6 ==
  In1 : Inport
  Integrator1 : Integrator
  Ws->kWh : Gain  Gain=1/3600/1000
  Out1 : Outport  VectorParamsAs1DForOutWhenUnconnected=off
  wires:
  Ws->kWh/1 -> Out1/1
  Integrator1/1 -> Ws->kWh/1
  In1/1 -> Integrator1/1

== system building_PHPP_v2/DATALOGGER/logger_BDB/z1/Subsystem7 ==
  In1 : Inport
  Integrator1 : Integrator
  Ws->kWh : Gain  Gain=1/3600/1000
  Out1 : Outport  VectorParamsAs1DForOutWhenUnconnected=off
  wires:
  In1/1 -> Integrator1/1
  Integrator1/1 -> Ws->kWh/1
  Ws->kWh/1 -> Out1/1

== system building_PHPP_v2/DATALOGGER/logger_BDB/z1/Subsystem8 ==
  In1 : Inport
  Integrator1 : Integrator
  Ws->kWh : Gain  Gain=1/3600/1000
  Out1 : Outport  VectorParamsAs1DForOutWhenUnconnected=off
  wires:
  Ws->kWh/1 -> Out1/1
  Integrator1/1 -> Ws->kWh/1
  In1/1 -> Integrator1/1

== system building_PHPP_v2/DATALOGGER/logger_BDB/z1/Subsystem9 ==
  In1 : Inport
  Integrator1 : Integrator
  Ws->kWh : Gain  Gain=1/3600/1000
  Out1 : Outport  VectorParamsAs1DForOutWhenUnconnected=off
  wires:
  In1/1 -> Integrator1/1
  Integrator1/1 -> Ws->kWh/1
  Ws->kWh/1 -> Out1/1

== system building_PHPP_v2/DATALOGGER/logger_BDB/z10/Subsystem ==
  In1 : Inport
  Integrator1 : Integrator
  Ws->kWh : Gain  Gain=1/3600/1000
  Out1 : Outport  VectorParamsAs1DForOutWhenUnconnected=off
  wires:
  In1/1 -> Integrator1/1
  Integrator1/1 -> Ws->kWh/1
  Ws->kWh/1 -> Out1/1

== system building_PHPP_v2/DATALOGGER/logger_BDB/z10/Subsystem1 ==
  In1 : Inport
  Integrator1 : Integrator
  Ws->kWh : Gain  Gain=1/3600/1000
  Out1 : Outport  VectorParamsAs1DForOutWhenUnconnected=off
  wires:
  Ws->kWh/1 -> Out1/1
  Integrator1/1 -> Ws->kWh/1
  In1/1 -> Integrator1/1

== system building_PHPP_v2/DATALOGGER/logger_BDB/z10/Subsystem10 ==
  In1 : Inport
  Integrator1 : Integrator
  Ws->kWh : Gain  Gain=1/3600/1000
  Out1 : Outport  VectorParamsAs1DForOutWhenUnconnected=off
  wires:
  In1/1 -> Integrator1/1
  Integrator1/1 -> Ws->kWh/1
  Ws->kWh/1 -> Out1/1

== system building_PHPP_v2/DATALOGGER/logger_BDB/z10/Subsystem11 ==
  In1 : Inport
  Integrator1 : Integrator
  Ws->kWh : Gain  Gain=1/3600/1000
  Out1 : Outport  VectorParamsAs1DForOutWhenUnconnected=off
  wires:
  Ws->kWh/1 -> Out1/1
  Integrator1/1 -> Ws->kWh/1
  In1/1 -> Integrator1/1

== system building_PHPP_v2/DATALOGGER/logger_BDB/z10/Subsystem12 ==
  In1 : Inport
  Integrator1 : Integrator
  Ws->kWh : Gain  Gain=1/3600/1000
  Out1 : Outport  VectorParamsAs1DForOutWhenUnconnected=off
  wires:
  In1/1 -> Integrator1/1
  Integrator1/1 -> Ws->kWh/1
  Ws->kWh/1 -> Out1/1

== system building_PHPP_v2/DATALOGGER/logger_BDB/z10/Subsystem2 ==
  In1 : Inport
  Integrator1 : Integrator
  Ws->kWh : Gain  Gain=1/3600/1000
  Out1 : Outport  VectorParamsAs1DForOutWhenUnconnected=off
  wires:
  In1/1 -> Integrator1/1
  Integrator1/1 -> Ws->kWh/1
  Ws->kWh/1 -> Out1/1

== system building_PHPP_v2/DATALOGGER/logger_BDB/z10/Subsystem3 ==
  In1 : Inport
  Integrator1 : Integrator
  Ws->kWh : Gain  Gain=1/3600/1000
  Out1 : Outport  VectorParamsAs1DForOutWhenUnconnected=off
  wires:
  Ws->kWh/1 -> Out1/1
  Integrator1/1 -> Ws->kWh/1
  In1/1 -> Integrator1/1

== system building_PHPP_v2/DATALOGGER/logger_BDB/z10/Subsystem4 ==
  In1 : Inport
  Integrator1 : Integrator
  Ws->kWh : Gain  Gain=1/3600/1000
  Out1 : Outport  VectorParamsAs1DForOutWhenUnconnected=off
  wires:
  In1/1 -> Integrator1/1
  Integrator1/1 -> Ws->kWh/1
  Ws->kWh/1 -> Out1/1

== system building_PHPP_v2/DATALOGGER/logger_BDB/z10/Subsystem5 ==
  In1 : Inport
  Integrator1 : Integrator
  Ws->kWh : Gain  Gain=1/3600/1000
  Out1 : Outport  VectorParamsAs1DForOutWhenUnconnected=off
  wires:
  Ws->kWh/1 -> Out1/1
  Integrator1/1 -> Ws->kWh/1
  In1/1 -> Integrator1/1

== system building_PHPP_v2/DATALOGGER/logger_BDB/z10/Subsystem6 ==
  In1 : Inport
  Integrator1 : Integrator
  Ws->kWh : Gain  Gain=1/3600/1000
  Out1 : Outport  VectorParamsAs1DForOutWhenUnconnected=off
  wires:
  In1/1 -> Integrator1/1
  Integrator1/1 -> Ws->kWh/1
  Ws->kWh/1 -> Out1/1

== system building_PHPP_v2/DATALOGGER/logger_BDB/z10/Subsystem7 ==
  In1 : Inport
  Integrator1 : Integrator
  Ws->kWh : Gain  Gain=1/3600/1000
  Out1 : Outport  VectorParamsAs1DForOutWhenUnconnected=off
  wires:
  Ws->kWh/1 -> Out1/1
  Integrator1/1 -> Ws->kWh/1
  In1/1 -> Integrator1/1

== system building_PHPP_v2/DATALOGGER/logger_BDB/z10/Subsystem8 ==
  In1 : Inport
  Integrator1 : Integrator
  Ws->kWh : Gain  Gain=1/3600/1000
  Out1 : Outport  VectorParamsAs1DForOutWhenUnconnected=off
  wires:
  In1/1 -> Integrator1/1
  Integrator1/1 -> Ws->kWh/1
  Ws->kWh/1 -> Out1/1

== system building_PHPP_v2/DATALOGGER/logger_BDB/z10/Subsystem9 ==
  In1 : Inport
  Integrator1 : Integrator
  Ws->kWh : Gain  Gain=1/3600/1000
  Out1 : Outport  VectorParamsAs1DForOutWhenUnconnected=off
  wires:
  Ws->kWh/1 -> Out1/1
  Integrator1/1 -> Ws->kWh/1
  In1/1 -> Integrator1/1

== system building_PHPP_v2/DATALOGGER/logger_BDB/z2/Subsystem ==
  In1 : Inport
  Integrator1 : Integrator
  Ws->kWh : Gain  Gain=1/3600/1000
  Out1 : Outport  VectorParamsAs1DForOutWhenUnconnected=off
  wires:
  In1/1 -> Integrator1/1
  Integrator1/1 -> Ws->kWh/1
  Ws->kWh/1 -> Out1/1

== system building_PHPP_v2/DATALOGGER/logger_BDB/z2/Subsystem1 ==
  In1 : Inport
  Integrator1 : Integrator
  Ws->kWh : Gain  Gain=1/3600/1000
  Out1 : Outport  VectorParamsAs1DForOutWhenUnconnected=off
  wires:
  Ws->kWh/1 -> Out1/1
  Integrator1/1 -> Ws->kWh/1
  In1/1 -> Integrator1/1

== system building_PHPP_v2/DATALOGGER/logger_BDB/z2/Subsystem10 ==
  In1 : Inport
  Integrator1 : Integrator
  Ws->kWh : Gain  Gain=1/3600/1000
  Out1 : Outport  VectorParamsAs1DForOutWhenUnconnected=off
  wires:
  In1/1 -> Integrator1/1
  Integrator1/1 -> Ws->kWh/1
  Ws->kWh/1 -> Out1/1

== system building_PHPP_v2/DATALOGGER/logger_BDB/z2/Subsystem11 ==
  In1 : Inport
  Integrator1 : Integrator
  Ws->kWh : Gain  Gain=1/3600/1000
  Out1 : Outport  VectorParamsAs1DForOutWhenUnconnected=off
  wires:
  Ws->kWh/1 -> Out1/1
  Integrator1/1 -> Ws->kWh/1
  In1/1 -> Integrator1/1

== system building_PHPP_v2/DATALOGGER/logger_BDB/z2/Subsystem12 ==
  In1 : Inport
  Integrator1 : Integrator
  Ws->kWh : Gain  Gain=1/3600/1000
  Out1 : Outport  VectorParamsAs1DForOutWhenUnconnected=off
  wires:
  In1/1 -> Integrator1/1
  Integrator1/1 -> Ws->kWh/1
  Ws->kWh/1 -> Out1/1

== system building_PHPP_v2/DATALOGGER/logger_BDB/z2/Subsystem2 ==
  In1 : Inport
  Integrator1 : Integrator
  Ws->kWh : Gain  Gain=1/3600/1000
  Out1 : Outport  VectorParamsAs1DForOutWhenUnconnected=off
  wires:
  In1/1 -> Integrator1/1
  Integrator1/1 -> Ws->kWh/1
  Ws->kWh/1 -> Out1/1

== system building_PHPP_v2/DATALOGGER/logger_BDB/z2/Subsystem3 ==
  In1 : Inport
  Integrator1 : Integrator
  Ws->kWh : Gain  Gain=1/3600/1000
  Out1 : Outport  VectorParamsAs1DForOutWhenUnconnected=off
  wires:
  Ws->kWh/1 -> Out1/1
  Integrator1/1 -> Ws->kWh/1
  In1/1 -> Integrator1/1

== system building_PHPP_v2/DATALOGGER/logger_BDB/z2/Subsystem4 ==
  In1 : Inport
  Integrator1 : Integrator
  Ws->kWh : Gain  Gain=1/3600/1000
  Out1 : Outport  VectorParamsAs1DForOutWhenUnconnected=off
  wires:
  In1/1 -> Integrator1/1
  Integrator1/1 -> Ws->kWh/1
  Ws->kWh/1 -> Out1/1

== system building_PHPP_v2/DATALOGGER/logger_BDB/z2/Subsystem5 ==
  In1 : Inport
  Integrator1 : Integrator
  Ws->kWh : Gain  Gain=1/3600/1000
  Out1 : Outport  VectorParamsAs1DForOutWhenUnconnected=off
  wires:
  Ws->kWh/1 -> Out1/1
  Integrator1/1 -> Ws->kWh/1
  In1/1 -> Integrator1/1

== system building_PHPP_v2/DATALOGGER/logger_BDB/z2/Subsystem6 ==
  In1 : Inport
  Integrator1 : Integrator
  Ws->kWh : Gain  Gain=1/3600/1000
  Out1 : Outport  VectorParamsAs1DForOutWhenUnconnected=off
  wires:
  In1/1 -> Integrator1/1
  Integrator1/1 -> Ws->kWh/1
  Ws->kWh/1 -> Out1/1

== system building_PHPP_v2/DATALOGGER/logger_BDB/z2/Subsystem7 ==
  In1 : Inport
  Integrator1 : Integrator
  Ws->kWh : Gain  Gain=1/3600/1000
  Out1 : Outport  VectorParamsAs1DForOutWhenUnconnected=off
  wires:
  Ws->kWh/1 -> Out1/1
  Integrator1/1 -> Ws->kWh/1
  In1/1 -> Integrator1/1

== system building_PHPP_v2/DATALOGGER/logger_BDB/z2/Subsystem8 ==
  In1 : Inport
  Integrator1 : Integrator
  Ws->kWh : Gain  Gain=1/3600/1000
  Out1 : Outport  VectorParamsAs1DForOutWhenUnconnected=off
  wires:
  In1/1 -> Integrator1/1
  Integrator1/1 -> Ws->kWh/1
  Ws->kWh/1 -> Out1/1

== system building_PHPP_v2/DATALOGGER/logger_BDB/z2/Subsystem9 ==
  In1 : Inport
  Integrator1 : Integrator
  Ws->kWh : Gain  Gain=1/3600/1000
  Out1 : Outport  VectorParamsAs1DForOutWhenUnconnected=off
  wires:
  Ws->kWh/1 -> Out1/1
  Integrator1/1 -> Ws->kWh/1
  In1/1 -> Integrator1/1

== system building_PHPP_v2/DATALOGGER/logger_BDB/z3/Subsystem ==
  In1 : Inport
  Integrator1 : Integrator
  Ws->kWh : Gain  Gain=1/3600/1000
  Out1 : Outport  VectorParamsAs1DForOutWhenUnconnected=off
  wires:
  Ws->kWh/1 -> Out1/1
  Integrator1/1 -> Ws->kWh/1
  In1/1 -> Integrator1/1

== system building_PHPP_v2/DATALOGGER/logger_BDB/z3/Subsystem1 ==
  In1 : Inport
  Integrator1 : Integrator
  Ws->kWh : Gain  Gain=1/3600/1000
  Out1 : Outport  VectorParamsAs1DForOutWhenUnconnected=off
  wires:
  In1/1 -> Integrator1/1
  Integrator1/1 -> Ws->kWh/1
  Ws->kWh/1 -> Out1/1

== system building_PHPP_v2/DATALOGGER/logger_BDB/z3/Subsystem10 ==
  In1 : Inport
  Integrator1 : Integrator
  Ws->kWh : Gain  Gain=1/3600/1000
  Out1 : Outport  VectorParamsAs1DForOutWhenUnconnected=off
  wires:
  Ws->kWh/1 -> Out1/1
  Integrator1/1 -> Ws->kWh/1
  In1/1 -> Integrator1/1

== system building_PHPP_v2/DATALOGGER/logger_BDB/z3/Subsystem11 ==
  In1 : Inport
  Integrator1 : Integrator
  Ws->kWh : Gain  Gain=1/3600/1000
  Out1 : Outport  VectorParamsAs1DForOutWhenUnconnected=off
  wires:
  In1/1 -> Integrator1/1
  Integrator1/1 -> Ws->kWh/1
  Ws->kWh/1 -> Out1/1

== system building_PHPP_v2/DATALOGGER/logger_BDB/z3/Subsystem12 ==
  In1 : Inport
  Integrator1 : Integrator
  Ws->kWh : Gain  Gain=1/3600/1000
  Out1 : Outport  VectorParamsAs1DForOutWhenUnconnected=off
  wires:
  Ws->kWh/1 -> Out1/1
  Integrator1/1 -> Ws->kWh/1
  In1/1 -> Integrator1/1

== system building_PHPP_v2/DATALOGGER/logger_BDB/z3/Subsystem2 ==
  In1 : Inport
  Integrator1 : Integrator
  Ws->kWh : Gain  Gain=1/3600/1000
  Out1 : Outport  VectorParamsAs1DForOutWhenUnconnected=off
  wires:
  Ws->kWh/1 -> Out1/1
  Integrator1/1 -> Ws->kWh/1
  In1/1 -> Integrator1/1

== system building_PHPP_v2/DATALOGGER/logger_BDB/z3/Subsystem3 ==
  In1 : Inport
  Integrator1 : Integrator
  Ws->kWh : Gain  Gain=1/3600/1000
  Out1 : Outport  VectorParamsAs1DForOutWhenUnconnected=off
  wires:
  In1/1 -> Integrator1/1
  Integrator1/1 -> Ws->kWh/1
  Ws->kWh/1 -> Out1/1

== system building_PHPP_v2/DATALOGGER/logger_BDB/z3/Subsystem4 ==
  In1 : Inport
  Integrator1 : Integrator
  Ws->kWh : Gain  Gain=1/3600/1000
  Out1 : Outport  VectorParamsAs1DForOutWhenUnconnected=off
  wires:
  Ws->kWh/1 -> Out1/1
  Integrator1/1 -> Ws->kWh/1
  In1/1 -> Integrator1/1

== system building_PHPP_v2/DATALOGGER/logger_BDB/z3/Subsystem5 ==
  In1 : Inport
  Integrator1 : Integrator
  Ws->kWh : Gain  Gain=1/3600/1000
  Out1 : Outport  VectorParamsAs1DForOutWhenUnconnected=off
  wires:
  In1/1 -> Integrator1/1
  Integrator1/1 -> Ws->kWh/1
  Ws->kWh/1 -> Out1/1

== system building_PHPP_v2/DATALOGGER/logger_BDB/z3/Subsystem6 ==
  In1 : Inport
  Integrator1 : Integrator
  Ws->kWh : Gain  Gain=1/3600/1000
  Out1 : Outport  VectorParamsAs1DForOutWhenUnconnected=off
  wires:
  Ws->kWh/1 -> Out1/1
  Integrator1/1 -> Ws->kWh/1
  In1/1 -> Integrator1/1

== system building_PHPP_v2/DATALOGGER/logger_BDB/z3/Subsystem7 ==
  In1 : Inport
  Integrator1 : Integrator
  Ws->kWh : Gain  Gain=1/3600/1000
  Out1 : Outport  VectorParamsAs1DForOutWhenUnconnected=off
  wires:
  In1/1 -> Integrator1/1
  Integrator1/1 -> Ws->kWh/1
  Ws->kWh/1 -> Out1/1

== system building_PHPP_v2/DATALOGGER/logger_BDB/z3/Subsystem8 ==
  In1 : Inport
  Integrator1 : Integrator
  Ws->kWh : Gain  Gain=1/3600/1000
  Out1 : Outport  VectorParamsAs1DForOutWhenUnconnected=off
  wires:
  Ws->kWh/1 -> Out1/1
  Integrator1/1 -> Ws->kWh/1
  In1/1 -> Integrator1/1

== system building_PHPP_v2/DATALOGGER/logger_BDB/z3/Subsystem9 ==
  In1 : Inport
  Integrator1 : Integrator
  Ws->kWh : Gain  Gain=1/3600/1000
  Out1 : Outport  VectorParamsAs1DForOutWhenUnconnected=off
  wires:
  In1/1 -> Integrator1/1
  Integrator1/1 -> Ws->kWh/1
  Ws->kWh/1 -> Out1/1

== system building_PHPP_v2/DATALOGGER/logger_BDB/z4/Subsystem ==
  In1 : Inport
  Integrator1 : Integrator
  Ws->kWh : Gain  Gain=1/3600/1000
  Out1 : Outport  VectorParamsAs1DForOutWhenUnconnected=off
  wires:
  In1/1 -> Integrator1/1
  Integrator1/1 -> Ws->kWh/1
  Ws->kWh/1 -> Out1/1

== system building_PHPP_v2/DATALOGGER/logger_BDB/z4/Subsystem1 ==
  In1 : Inport
  Integrator1 : Integrator
  Ws->kWh : Gain  Gain=1/3600/1000
  Out1 : Outport  VectorParamsAs1DForOutWhenUnconnected=off
  wires:
  Ws->kWh/1 -> Out1/1
  Integrator1/1 -> Ws->kWh/1
  In1/1 -> Integrator1/1

== system building_PHPP_v2/DATALOGGER/logger_BDB/z4/Subsystem10 ==
  In1 : Inport
  Integrator1 : Integrator
  Ws->kWh : Gain  Gain=1/3600/1000
  Out1 : Outport  VectorParamsAs1DForOutWhenUnconnected=off
  wires:
  In1/1 -> Integrator1/1
  Integrator1/1 -> Ws->kWh/1
  Ws->kWh/1 -> Out1/1
